simulink model "ThreeDOF_Rocket_Simulator_v2_CL"  (R2023b)
settings: Solver=VariableStepAuto  StartTime=0.0  StopTime=53  RelTol=1e-3
libraries: shared3dof x1
settings Model: Creator=giuse  LastModifiedBy=giuse
settings OptimizationCC: ReuseModelBlockBuffer=off
settings DebuggingCC: UnconnectedInputMsg=warning  UnconnectedOutputMsg=warning  UnconnectedLineMsg=warning
settings ModelReferenceCC: EnableRefExpFcnMdlSchedulingChecks=on
settings RTWCC: DLArmComputeVersion=19.05

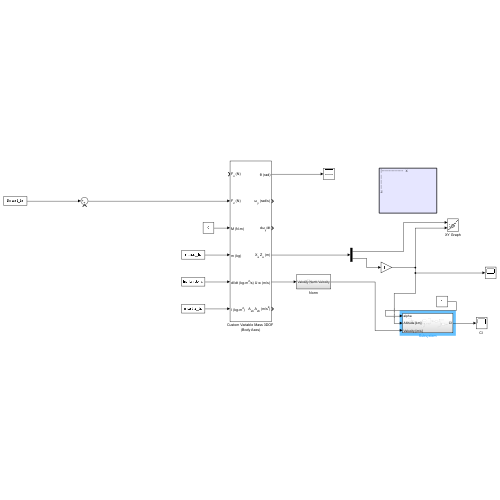
[thumbnail: Simulink's stored preview of the top-level diagram]
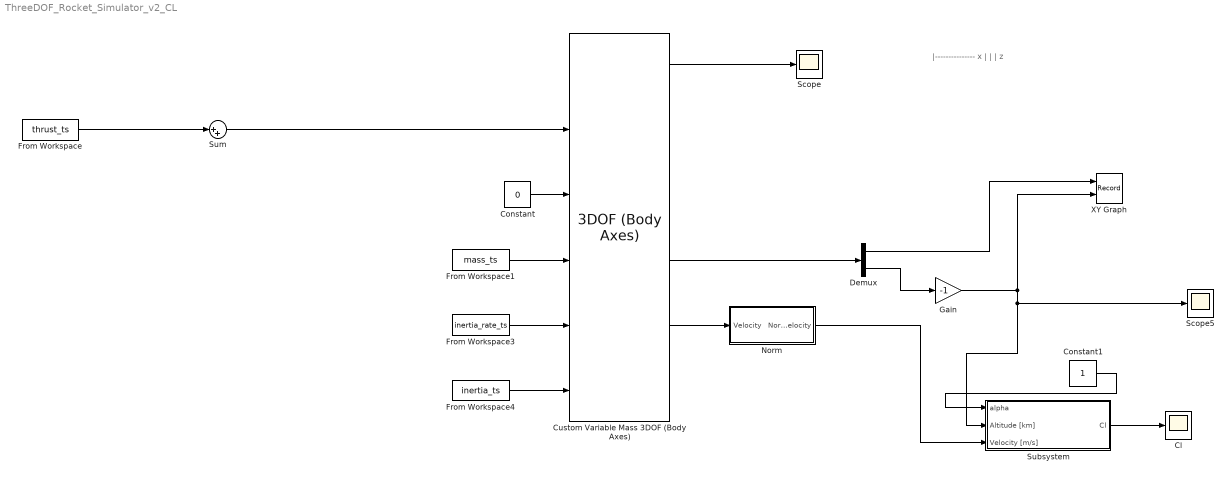
== system ThreeDOF_Rocket_Simulator_v2_CL ==
  note: |---------------  x
      | |
      | |
      | |
      | z
  "Cl " : Scope
  Constant : Constant  Value=0
  Constant1 : Constant
  Custom Variable Mass 3DOF (Body Axes) : shared3dof/3DOF (Body Axes)  units=Metric (MKS)  mtype=Custom Variable  v_ini=0  theta_ini=pi  alpha_ini=0  pos_ini=[0 0]  q_ini=0  mass=1.0  mass_e=0.5  mass_f=3.0  Iyy=1.0  Iyy_e=0.5  Iyy_f=3.0  g_in=Internal  g=9.81  vre_flag=off  abi_flag=off  aMode=0  vel_statename=''  theta_statename=''  pos_statename=''  q_statename=''  mass_statename=''
  Demux : Demux  Outputs=2
  From Workspace : FromWorkspace  VariableName=thrust_ts
  From Workspace1 : FromWorkspace  VariableName=mass_ts
  From Workspace3 : FromWorkspace  VariableName=inertia_rate_ts
  From Workspace4 : FromWorkspace  VariableName=inertia_ts
  Gain : Gain  Gain=-1
  Norm : Subsystem
  Scope : Scope
  Scope5 : Scope
  Subsystem : Subsystem
  Sum : Sum  Inputs=|++
  XY Graph : Record  FileSettingsInternal="{\"entries\":[{\"content\":{\"excelSettings\":{\"content\":{},\"type\":\"Streamout.ExcelSettings\"}},\"type\":\"Streamout.FileSettingStorage\",\"uuid\":\"\"}],\"packageUris\":[\"http:\\/\\/schema.mathworks.com\\/mf0\\/streamout_blocks\\/R2020a\"],\"version\":\"1.0\"}"  Layout=[1 1]  SignalsInternal="{\"entries\":[{\"content\":{\"signals\":[{\"content\":{\"blockPath\":[],\"dimensions\":[1],\"domain\":\"\",\"lineColor\":\"#a2142f\",\"plots\":[1],\"port\":1,\"signalID\":8,\"signalName\":\"Demux:1\"},\"type\":\"RecordBlkView.Signal\",\"uuid\":\"\"},{\"content\":{\"blockPath\":[],\"dimensions\":[1],\"domain\":\"\",\"lineColor\":\"#139fff\",\"plots\":[1],\"port\":2,\"signalID\":11,\"signalName\":\"Gain\"},\"type\":\"RecordBlkView.Signal\",\"uuid\":\"\"}]},\"type\":\"RecordBlkView.InputSignals\",\"uuid\":\"\"}],\"packageUris\":[\"http:\\/\\/schema.mathworks.com\\/mf0\\/streamout_blocks\\/R2020a\"],\"version\":\"1.0\"}"  VisualizationBindings="{\"xyplotplugin\":{\"info\":[{\"series\":[{\"bindingParametersList\":[{\"parameter\":\"Y-Axis\",\"signalID\":11,\"signalName\":\"Gain\"},{\"parameter\":\"X-Axis\",\"signalID\":8,\"signalName\":\"Demux:1\"}],\"seriesID\":51063}],\"subplotID\":1}]}}"  CompatibilityTag=XY  st=-1
  wires:
  From Workspace1/1 -> Custom Variable Mass 3DOF (Body Axes)/4
  From Workspace3/1 -> Custom Variable Mass 3DOF (Body Axes)/5
  From Workspace4/1 -> Custom Variable Mass 3DOF (Body Axes)/6
  Demux/2 -> Gain/1
  Demux/1 -> XY Graph/1
  Custom Variable Mass 3DOF (Body Axes)/4 -> Demux/1
  From Workspace/1 -> Sum/1
  Sum/1 -> Custom Variable Mass 3DOF (Body Axes)/2
  Custom Variable Mass 3DOF (Body Axes)/1 -> Scope/1
  Constant/1 -> Custom Variable Mass 3DOF (Body Axes)/3
  Subsystem/1(Cl) -> "Cl "/1
  Custom Variable Mass 3DOF (Body Axes)/5 -> Norm/1(Velocity)
  Norm/1(Norm Velocity) -> Subsystem/3(Velocity [m/s])
  Gain/1 -> Subsystem/2(Altitude [km]), Scope5/1, XY Graph/2
  Constant1/1 -> Subsystem/1(alpha)

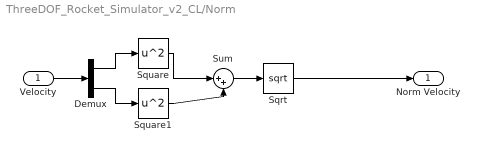
== system ThreeDOF_Rocket_Simulator_v2_CL/Norm ==
  Velocity : Inport
  Demux : Demux  Outputs=2
  Sqrt : Sqrt
  Square : Math  Operator=square
  Square1 : Math  Operator=square
  Sum : Sum  Inputs=|++
  Norm Velocity : Outport
  wires:
  Square/1 -> Sum/1
  Square1/1 -> Sum/2
  Sum/1 -> Sqrt/1
  Sqrt/1 -> Norm Velocity/1
  Demux/1 -> Square/1
  Demux/2 -> Square1/1
  Velocity/1 -> Demux/1

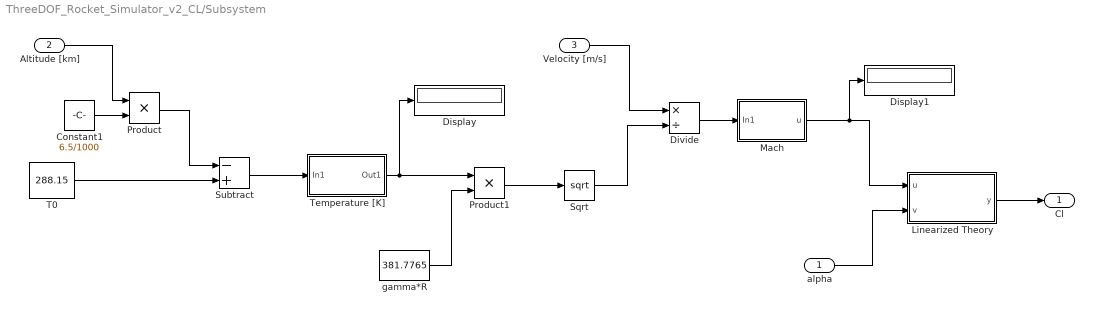
== system ThreeDOF_Rocket_Simulator_v2_CL/Subsystem ==
  alpha : Inport
  Altitude [km] : Inport  Port=2
  Velocity [m/s] : Inport  Port=3
  Constant1 : Constant  Value=6.5/1000
  Display : Display
  Display1 : Display
  Divide : Product  Inputs=*/
  Linearized Theory : MATLAB Function  TreatAsAtomicUnit=on
  Mach : Subsystem
  Product : Product
  Product1 : Product
  Sqrt : Sqrt
  Subtract : Sum  Inputs=-+
  T0 : Constant  Value=288.15
  Temperature [K] : Subsystem
  gamma*R : Constant  Value=381.7765
  Cl : Outport
  wires:
  Constant1/1 -> Product/2
  Temperature [K]/1(Out1) -> Display/1, Product1/1
  T0/1 -> Subtract/2
  Subtract/1 -> Temperature [K]/1(In1)
  Mach/1(u) -> Display1/1, Linearized Theory/1(u)
  Divide/1 -> Mach/1(In1)
  Sqrt/1 -> Divide/2
  Product/1 -> Subtract/1
  gamma*R/1 -> Product1/2
  Velocity [m/s]/1 -> Divide/1
  Product1/1 -> Sqrt/1
  alpha/1 -> Linearized Theory/2(v)
  Linearized Theory/1(y) -> Cl/1
  Altitude [km]/1 -> Product/1

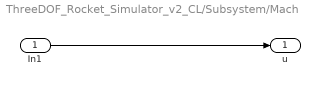
== system ThreeDOF_Rocket_Simulator_v2_CL/Subsystem/Mach ==
  In1 : Inport
  u : Outport
  wires:
  In1/1 -> u/1

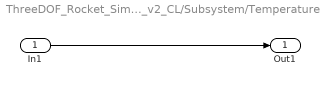
== system ThreeDOF_Rocket_Simulator_v2_CL/Subsystem/Temperature [K] ==
  In1 : Inport
  Out1 : Outport
  wires:
  In1/1 -> Out1/1

== matlab function ThreeDOF_Rocket_Simulator_v2_CL/Subsystem/Linearized Theory ==
  data: u input; y output; v input
function y = fcn(u,v)
% First method, linearized theory for a thin plate
if u<1
    y = ((2*pi*(v*2*pi)/360)./(sqrt(1-u.^2)))*13500/(2*pi*52^2).*2;
else
    y= 4*(4*(v*pi/180))./(sqrt(u^2-1)+2*(v*pi/180))

end
